simulink model "Good_Maglev_PI_Control"  (R2023b)
settings: Solver=VariableStepAuto  StartTime=0.0  StopTime=10.0  RelTol=1e-3
settings Model: Creator=cyrus  LastModifiedBy=cyrus

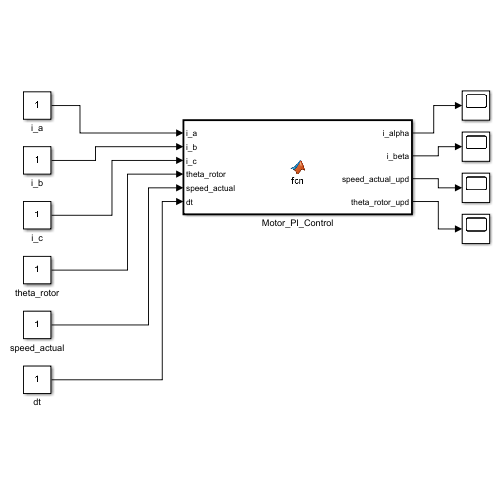
[thumbnail: Simulink's stored preview of the top-level diagram]
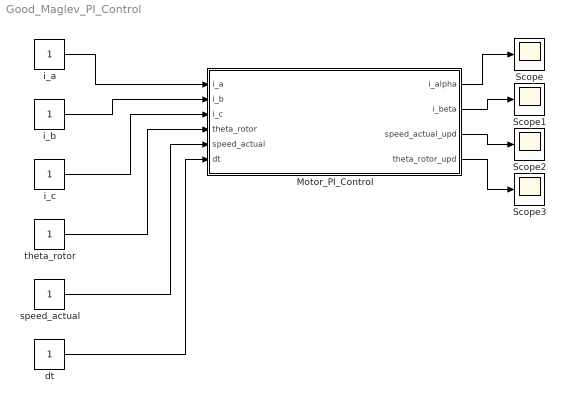
== system Good_Maglev_PI_Control ==
  Motor_PI_Control : MATLAB Function  TreatAsAtomicUnit=on
  Scope{,1..3} (4 alike) : Scope
  dt : Constant
  i_a : Constant
  i_b : Constant
  i_c : Constant
  speed_actual : Constant
  theta_rotor : Constant
  wires:
  i_a/1 -> Motor_PI_Control/1(i_a)
  i_b/1 -> Motor_PI_Control/2(i_b)
  i_c/1 -> Motor_PI_Control/3(i_c)
  theta_rotor/1 -> Motor_PI_Control/4(theta_rotor)
  speed_actual/1 -> Motor_PI_Control/5(speed_actual)
  Motor_PI_Control/1(i_alpha) -> Scope/1
  Motor_PI_Control/2(i_beta) -> Scope1/1
  dt/1 -> Motor_PI_Control/6(dt)
  Motor_PI_Control/3(speed_actual_upd) -> Scope2/1
  Motor_PI_Control/4(theta_rotor_upd) -> Scope3/1

== matlab function Good_Maglev_PI_Control/Motor_PI_Control ==
  data: i_a input; i_alpha output; i_b input; i_c input; theta_rotor input; speed_actual input; i_beta output; speed_actual_upd output; theta_rotor_upd output; dt input
function [i_alpha, i_beta, speed_actual_upd, theta_rotor_upd] = ...
    fcn(i_a, i_b, i_c, theta_rotor, speed_actual, dt)
% fcn: Combined controller + simple motor plant
%
% Inputs:
%   i_a, i_b, i_c     : Three-phase currents (A)
%   theta_rotor       : Rotor angle (rad)
%   speed_actual      : Motor speed (rpm)
%   dt                : Simulation time step (s)
%
% Outputs:
%   i_alpha, i_beta   : Stationary frame currents from the controller (A)
%   speed_actual_upd  : Updated motor speed (rpm)
%   theta_rotor_upd   : Updated rotor angle (rad)

    %% 1) Controller Parameters
    KPq = 1.0;   KIq = 0.1;
    KPd = 1.0;   KId = 0.1;

    SPEED_REF = 1000.0;   % Desired speed (rpm)
    id_ref    = 0;        % Flux reference

    % Persistent integrators
    persistent integral_error_q integral_error_d
    if isempty(integral_error_q)
        integral_error_q = 0.0;
    end
    if isempty(integral_error_d)
        integral_error_d = 0.0;
    end

    %% 2) Controller: Clarke Transform (3-phase -> alpha-beta)
    i_alpha_temp = (2/3)*( i_a - 0.5*i_b - 0.5*i_c );
    i_beta_temp  = (2/3)*((sqrt(3)/2)*( i_b - i_c ));

    %% 3) Controller: Park Transform (alpha-beta -> d-q)
    i_d =  i_alpha_temp*cos(theta_rotor) + i_beta_temp*sin(theta_rotor);
    i_q = -i_alpha_temp*sin(theta_rotor) + i_beta_temp*cos(theta_rotor);

    %% 4) Speed PI control (affects i_q)
    speed_error       = SPEED_REF - speed_actual;
    integral_error_q  = integral_error_q + speed_error*dt;  % multiply by dt for discrete integration
    i_q_new           = KPq * speed_error + KIq * integral_error_q;

    %% 5) Flux PI control (maintains i_d near id_ref)
    id_error          = id_ref - i_d;
    integral_error_d  = integral_error_d + id_error*dt;     % multiply by dt
    i_d_new           = KPd * id_error + KId * integral_error_d;

    %% 6) Controller: Inverse Park (d-q -> alpha-beta)
    i_alpha = i_d_new*cos(theta_rotor) - i_q_new*sin(theta_rotor);
    i_beta  = i_d_new*sin(theta_rotor) + i_q_new*cos(theta_rotor);

    %% 7) Plant: Simple Motor Dynamics
    % Parameters
    J  = 0.01;    % Inertia (kg*m^2)
    B  = 0.001;   % Damping (N*m/(rad/s))
    Kt = 0.1;     % Torque constant (N*m/A)

    % Convert speed from rpm to rad/s
    speed_rad = speed_actual * (2*pi/60);

    % Compute torque-producing current (i_q) from i_alpha, i_beta
    %   i_q = -alpha*sin(theta) + beta*cos(theta)
    i_q_plant = -i_alpha*sin(theta_rotor) + i_beta*cos(theta_rotor);

    % Motor torque
    torque = Kt * i_q_plant;

    % Equation of motion: d(omega)/dt = (torque - B*omega)/J
    acceleration    = (torque - B*speed_rad)/J;
    speed_rad       = speed_rad + acceleration * dt;
    theta_rotor_upd = theta_rotor + speed_rad * dt;

    % Convert speed back to rpm
    speed_actual_upd = speed_rad * (60/(2*pi));
end
